simulink model "chassis_passive_sim"  (R2014b)
settings: Solver=ode3  SolverMode=SingleTasking  StartTime=0.0  StopTime=run_time  FixedStep=0.001  RelTol=1e-3
values from neighbouring files (symbols this model uses):
  A = [0 1 0 0 ... (first row only)    [H_inf_ctrl.m]    (also in Hinf_control.m; TwoDOF_mat.m; chassis_passive.m; chassis_skyhook.m)
  B = [0 0 0 0 ... (first row only)    [H_inf_ctrl.m]    (also in Hinf_control.m; TwoDOF_mat.m = [0 0 0; chassis_passive.m; chassis_skyhook.m)
  C = [1 0 0 0 ... (first row only)    [H_inf_ctrl.m]    (also in Hinf_control.m; TwoDOF_mat.m = [1 0 0 0]; chassis_passive.m; chassis_skyhook.m)
  D = [0 0 0 0 ... (first row only)    [H_inf_ctrl.m]    (also in Hinf_control.m; TwoDOF_mat.m = [0 0 0]; chassis_passive.m; chassis_skyhook.m)
  exictation = 1    [H_inf_ctrl.m]    (also in Hinf_control.m = 0; chassis_passive.m = 0; chassis_skyhook.m)
  f = 1    [H_inf_ctrl.m]    (also in Hinf_control.m = 1.1792; chassis_passive.m = 8; chassis_skyhook.m = 1.1792)
settings Model: Creator=signat  LastModifiedBy=eric
settings OptimizationCC: BlockReduction=off  BooleanDataType=off
settings DebuggingCC: SaveWithParameterizedLinksMsg=none  UnderspecifiedInitializationDetection=Classic  MergeDetectMultiDrivingBlocksExec=none  SignalResolutionControl=TryResolveAllWithWarning  SolverPrmCheckMsg=none
settings HardwareCC: TargetUnknown=on

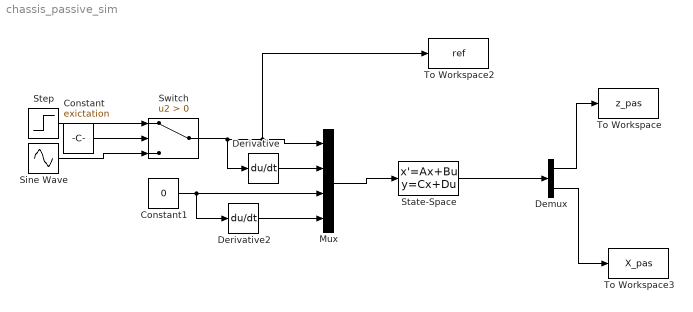
== system chassis_passive_sim ==
  Constant : Constant  Value=exictation
  Constant1 : Constant  Value=0
  Demux : Demux  Outputs=2
  Derivative : Derivative
  Derivative2 : Derivative
  Mux : Mux
  Sine Wave : Sin  Amplitude=0.01  Frequency=f*2*pi  SampleTime=0
  State-Space : StateSpace  A=A  B=B  C=C  D=D  X0=0
  Step : Step  After=0.03  SampleTime=0
  Switch : Switch  Criteria=u2 > Threshold
  To Workspace : ToWorkspace  VariableName=z_pas  SaveFormat=Timeseries  SampleTime=-1
  To Workspace2 : ToWorkspace  VariableName=ref  SaveFormat=Timeseries  SampleTime=-1
  To Workspace3 : ToWorkspace  VariableName=X_pas  SaveFormat=Timeseries  SampleTime=-1
  wires:
  Step/1 -> Switch/1
  Sine Wave/1 -> Switch/3
  Constant/1 -> Switch/2
  Derivative/1 -> Mux/2
  Mux/1 -> State-Space/1
  Switch/1 -> Derivative/1, To Workspace2/1, Mux/1
  Constant1/1 -> Derivative2/1, Mux/3
  Derivative2/1 -> Mux/4
  State-Space/1 -> Demux/1
  Demux/1 -> To Workspace/1
  Demux/2 -> To Workspace3/1
